simulink model "ext_loop"  (R2022a)
settings: Solver=VariableStepAuto  StartTime=0.0  StopTime=10.0  RelTol=1e-3
undefined symbols (not defined in the file or in its folder): P_ref
libraries: cstblocks x2
settings Model: Creator=fcampreg  LastModifiedBy=fcampreg

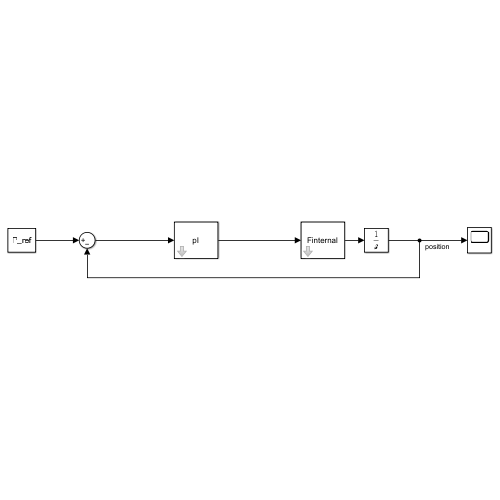
[thumbnail: Simulink's stored preview of the top-level diagram]
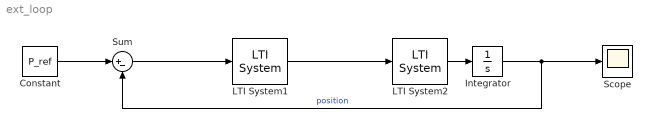
== system ext_loop ==
  Constant : Constant  Value=P_ref
  Integrator : Integrator
  LTI System1 : cstblocks/LTI System  sys=pI  IC=[]
  LTI System2 : cstblocks/LTI System  sys=Finternal  IC=[]
  Scope : Scope
  Sum : Sum  Inputs=|+-
  wires:
  LTI System1/1 -> LTI System2/1
  LTI System2/1 -> Integrator/1
  Sum/1 -> LTI System1/1
  Constant/1 -> Sum/1
  Integrator/1 -> Scope/1, Sum/2  "position"
